simulink model "Tape"  (R2025b)
settings: Solver=VariableStepAuto  StartTime=0.0  StopTime=0.5  RelTol=1e-3
values from neighbouring files (symbols this model uses):
  B = 20    [System_Parameters.m]
  B1 = 1e-2    (= 0.01)    [System_Parameters.m]
  B2 = 2e-2    (= 0.02)    [System_Parameters.m]
  J1 = 5e-5    (= 5e-05)    [System_Parameters.m]
  J2 = 2e-5    (= 2e-05)    [System_Parameters.m]
  K = 2e4    (= 20000)    [System_Parameters.m]
  Kt = 3e-2    (= 0.03)    [System_Parameters.m]
  r1 = 2e-2    (= 0.02)    [System_Parameters.m]
  r2 = 2e-2    (= 0.02)    [System_Parameters.m]
settings Model: Creator=AsusIran  LastModifiedBy=AsusIran
settings DebuggingCC: AlgebraicLoopMsg=none

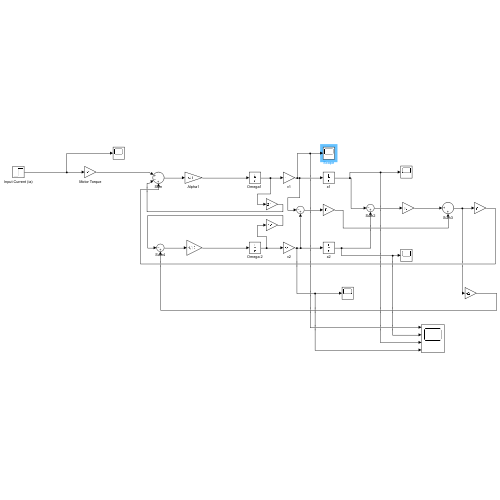
[thumbnail: Simulink's stored preview of the top-level diagram]
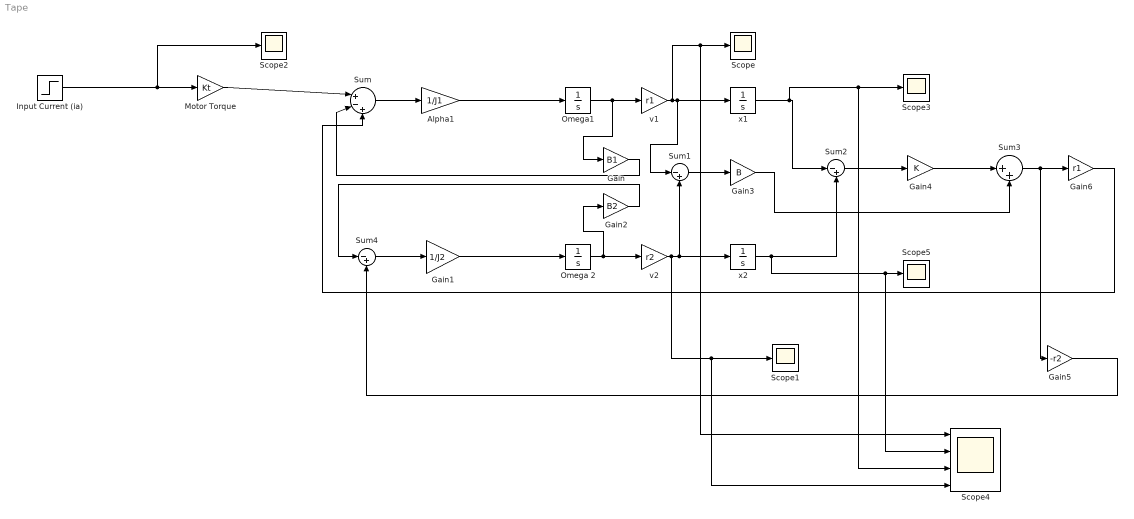
== system Tape ==
  Alpha1 : Gain  Gain=1/J1
  Gain : Gain  Gain=B1
  Gain1 : Gain  Gain=1/J2
  Gain2 : Gain  Gain=B2
  Gain3 : Gain  Gain=B
  Gain4 : Gain  Gain=K
  Gain5 : Gain  Gain=-r2
  Gain6 : Gain  Gain=r1
  Input Current (ia) : Step  Time=0  SampleTime=0
  Motor Torque : Gain  Gain=Kt
  Omega 2 : Integrator
  "Omega1 " : Integrator
  Scope{,1..3,5} (5 alike) : Scope
      Scope settings: ActiveDisplayYMinimum=0.010572480880899869  ActiveDisplayYMaximum=0.023213839605589589
      Scope1 settings: ActiveDisplayYMinimum=-0.0025468844121825621  ActiveDisplayYMaximum=0.022921959709643062
      Scope2 settings: ActiveDisplayYMinimum=-1  ActiveDisplayYMaximum=1  DataLoggingVariableName=ScopeData2
      Scope3 settings: ActiveDisplayYMinimum=-0.0012483333333333333  ActiveDisplayYMaximum=0.011235000000000002  DataLoggingVariableName=ScopeData3
      Scope5 settings: ActiveDisplayYMinimum=-0.0025468844121825621  ActiveDisplayYMaximum=0.022921959709643062  DataLoggingVariableName=ScopeData5
  Scope4 : Scope  NumInputPorts=4
      settings: ActiveDisplayYMinimum=-0.002759450072274548  ActiveDisplayYMaximum=0.024835050650470935  DataLoggingVariableName=ScopeData4
  Sum : Sum  Inputs=|+-+
  Sum1 : Sum  Inputs=|-+
  Sum2 : Sum  Inputs=|-+
  Sum3 : Sum  Inputs=|++
  Sum4 : Sum  Inputs=|-+
  v1 : Gain  Gain=r1
  v2 : Gain  Gain=r2
  x1 : Integrator
  x2 : Integrator  IgnoreLimit=on
  wires:
  Input Current (ia)/1 -> Scope2/1, Motor Torque/1
  Motor Torque/1 -> Sum/1
  Sum/1 -> Alpha1/1
  Alpha1/1 -> "Omega1 "/1
  "Omega1 "/1 -> Gain/1, v1/1
  v1/1 -> Scope4/1, Scope/1, Sum1/1, x1/1
  Sum4/1 -> Gain1/1
  Gain1/1 -> Omega 2/1
  Omega 2/1 -> Gain2/1, v2/1
  v2/1 -> Scope4/4, Scope1/1, Sum1/2, x2/1
  Sum1/1 -> Gain3/1
  x1/1 -> Scope4/3, Scope3/1, Sum2/1
  x2/1 -> Scope4/2, Scope5/1, Sum2/2
  Sum2/1 -> Gain4/1
  Gain4/1 -> Sum3/1
  Gain3/1 -> Sum3/2
  Sum3/1 -> Gain5/1, Gain6/1
  Gain6/1 -> Sum/3
  Gain/1 -> Sum/2
  Gain2/1 -> Sum4/1
  Gain5/1 -> Sum4/2
